simulink library "NetworksLib"  (Simulink 7.5)
settings: Solver=ode45  SolverMode=SingleTasking  StartTime=0.0  StopTime=10.0  RelTol=1e-3
undefined symbols (not defined in the file or in its folder): Others, SF, Sigmoid, to
libraries: simulink x3, NetworksLib x3, RateBasedLib x2, fuzblock x1, StimuliLib x1
settings Model: Creator=jpalma  LastModifiedBy=jpalma

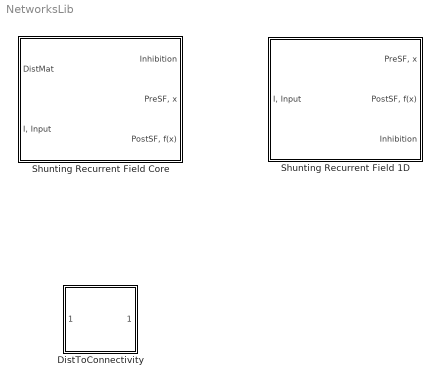
== system NetworksLib ==
  DistToConnectivity : Subsystem  mask{connectChoice=1-to-1, gaussWidth=1, gaussMean=0}
      mask prompts: gaussWidth "Gaussian Width"; gaussMean "Gaussian Mean"
      mask StyleString: popup(1-to-1|1-to-All|1-to-Others|Gaussian),edit,edit
      mask CallbackString:
      | maskStr = get_param(gcb,'MaskValues');
      | visibilitiesStr = {'on';'off';'off'};
      | if strcmp(maskStr{1},'Gaussian')
      |         visibilitiesStr(2) = {'on'};
      |         visibilitiesStr(3) = {'on'};
      | end
      | set_param(gcb,'MaskVisibilities',visibilitiesStr);||
      mask Display: image(imread('../libs/icons/Connect.jpg'),'center');
  Shunting Recurrent Field 1D : Subsystem  mask{signalFunction=Sigmoid-SF, threshold=0.3, thresholdSwitch=0, slope=9, asymptote=1, ground=0, A=0.1, B=1, fieldLength=10, ifCyclic=off, C=1, D=1, tau=1, inhibConnect=1-to-Others, inhibWidth=5, excitConnect=1-to-1, excitWidth=2}
      mask prompts: signalFunction "Signal Function Choice"; threshold "Threshold (SF)"; thresholdSwitch "Threshold of Switch (SF)"; slope "Slope (SF)"; asymptote "Asymptote (SF)"; ground "Ground (SF)"; A "A, Neuron Decay"; B "B, Neuron Shunting Max"; fieldLength "Field Length"; ifCyclic "Cyclic?"; C "C, Inhibitory Strength"; D "D, Excitatory Strength"; tau "tau, Time Constant"; inhibConnect "Inhibitory Connectivity"; inhibWidth "Inhibitory Width"; excitConnect "Excitatory Connectectivity"; excitWidth "Excitatory Width"
      mask init:
      | set_param([gcb '/Shunting Recurrent Field Core'], 'signalFunction', signalFunction);
      | set_param([gcb '/Shunting Recurrent Field Core'], 'threshold', threshold);
      | set_param([gcb '/Shunting Recurrent Field Core'], 'thresholdSwitch', thresholdSwitch);
      | set_param([gcb '/Shunting Recurrent Field Core'], 'slope', slope);
      | set_param([gcb '/Shunting Recurrent Field Core'], 'asymptote', asymptote);
      | set_param([gcb '/Shunting Recurrent Field Core'], 'ground', ground);
      | set_param([gcb '/Shunting Recurrent Field Core'], 'A', A);
      | set_param([gcb '/Shunting Recurrent Field Core'], 'B', B);
      | set_param([gcb '/Shunting Recurrent Field Core'], 'C', C);
      | set_param([gcb '/Shunting Recurrent Field Core'], 'D', D);
      | set_param([gcb '/Shunting Recurrent Field Core'], 'tau', tau);
      | set_param([gcb '/Shunting Recurrent Field Core'], 'inhibConnect', inhibConnect);
      | set_param([gcb '/Shunting Recurrent Field Core'], 'inhibWidth', inhibWidth);
      | set_param([gcb '/Shunting Recurrent Field Core'], 'excitConnect', excitConnect);
      | set_param([gcb '/Shunting Recurrent Field Core'], 'excitWidth', excitWidth);
      | set_param([gcb '/DistMatrix1D'], 'vectorLength', fieldLength);
      | set_param([gcb '/DistMatrix1D'], 'ifCyclic', ifCyclic);
      mask StyleString: popup(Linear-SF|Faster-SF|Slower-SF|Sigmoid-SF|Sigmoid-To-Linear-SF),edit,edit,edit,edit,edit,edit,edit,edit,checkbox,edit,edit,edit,popup(1-to-1|1-to-All|1-to-Others|Gaussian),edit,popup(1-to-1|1-to-All|1-to-Others|Gaussian),edit
      mask CallbackString:
      | maskStr = get_param(gcb,'MaskValues');
      | 
      | visibilitiesStr = {'on';'off';'off';'off';'off';'off';'on';'on'; ...
      |                    'on';'on';'on';'on';'on';'on';'off';'on';'off'};
      | if strcmp(maskStr{1},'Sigmoid-SF')
      |         visibilitiesStr(2) = {'on'};
      |         visibilitiesStr(4) = {'on'};
      |         visibilitiesStr(5) = {'on'};
      |         visibilitiesStr(6) = {'on'};
      | else if strcmp(maskStr{1},'Sigmoid-To-Linear-SF')
      |         visibilitiesStr(2) = {'on'};
      |         visibilitiesStr(3) = {'on'};
      |         visibilitiesStr(4) = {'on'};
      |         visibilitiesStr(5) = {'on'};
      |         visibilitiesStr(6) = {'on'};
      |     end
      | end
      | if strcmp(maskStr{14},'Gaussian')
      |         visibilitiesStr(15) = {'on'};
      | end
      | if strcmp(maskStr{16},'Gaussian')
      |         visibilitiesStr(17) = {'on'};
      | end
      | set_param(gcb,'MaskVisibilities',visibilitiesStr);
      | |||||||||||||maskStr = get_param(gcb,'MaskValues');
      | 
      | visibilitiesStr = {'on';'off';'off';'off';'off';'off';'on';'on'; ...
      |                    'on';'on';'on';'on';'on';'on';'off';'on';'off'};
      | if strcmp(maskStr{1},'Sigmoid-SF')
      |         visibilitiesStr(2) = {'on'};
      |         visibilitiesStr(4) = {'on'};
      |         visibilitiesStr(5) = {'on'};
      |         visibilitiesStr(6) = {'on'};
      | else if strcmp(maskStr{1},'Sigmoid-To-Linear-SF')
      |         visibilitiesStr(2) = {'on'};
      |         visibilitiesStr(3) = {'on'};
      |         visibilitiesStr(4) = {'on'};
      |         visibilitiesStr(5) = {'on'};
      |         visibilitiesStr(6) = {'on'};
      |     end
      | end
      | if strcmp(maskStr{14},'Gaussian')
      |         visibilitiesStr(15) = {'on'};
      | end
      | if strcmp(maskStr{16},'Gaussian')
      |         visibilitiesStr(17) = {'on'};
      | end
      | set_param(gcb,'MaskVisibilities',visibilitiesStr);||maskStr = get_param(gcb,'MaskValues');
      | 
      | visibilitiesStr = {'on';'off';'off';'off';'off';'off';'on';'on'; ...
      |                    'on';'on';'on';'on';'on';'on';'off';'on';'off'};
      | if strcmp(maskStr{1},'Sigmoid-SF')
      |         visibilitiesStr(2) = {'on'};
      |         visibilitiesStr(4) = {'on'};
      |         visibilitiesStr(5) = {'on'};
      |         visibilitiesStr(6) = {'on'};
      | else if strcmp(maskStr{1},'Sigmoid-To-Linear-SF')
      |         visibilitiesStr(2) = {'on'};
      |         visibilitiesStr(3) = {'on'};
      |         visibilitiesStr(4) = {'on'};
      |         visibilitiesStr(5) = {'on'};
      |         visibilitiesStr(6) = {'on'};
      |     end
      | end
      | if strcmp(maskStr{14},'Gaussian')
      |         visibilitiesStr(15) = {'on'};
      | end
      | if strcmp(maskStr{16},'Gaussian')
      |         visibilitiesStr(17) = {'on'};
      | end
      | set_param(gcb,'MaskVisibilities',visibilitiesStr);|
      mask Display: image(imread('../libs/icons/Networks.jpg'),'center');
  Shunting Recurrent Field Core : Subsystem  mask{signalFunction=Sigmoid-SF, threshold=0.3, thresholdSwitch=0, slope=9, asymptote=1, ground=0, A=0.1, B=1, C=1, D=1, tau=1, inhibConnect=1-to-Others, inhibWidth=5, excitConnect=1-to-1, excitWidth=2}
      mask prompts: signalFunction "Signal Function Choice"; threshold "Threshold (SF)"; thresholdSwitch "Threshold of Switch (SF)"; slope "Slope (SF)"; asymptote "Asymptote (SF)"; ground "Gound (SF)"; A "A, Neuron Decay"; B "B, Neuron Shunting Max"; C "C, Inhibitory Strength"; D "D, Excitatory Strength"; tau "tau, Time Constant"; inhibConnect "Inhibitory Connectivity"; inhibWidth "Inhibitory Width"; excitConnect "Excitatory Connectivity"; excitWidth "Excitatory Width"
      mask init:
      | set_param([gcb '/Signal Function'], 'BlockChoice', signalFunction);
      | if(strcmp(signalFunction,'Sigmoid-SF'))
      |    maskStr = get_param([gcb '/Signal Function/' signalFunction],'MaskValues');
      |    maskStr{1} = threshold;
      |    maskStr{2} = slope;
      |    maskStr{3} = asymptote;
      |    maskStr{4} = ground;
      |    set_param([gcb '/Signal Function/' signalFunction], 'MaskValues', maskStr);
      | end
      | if(strcmp(signalFunction,'Sigmoid-To-Linear-SF'))
      |    maskStr = get_param([gcb '/Signal Function/' signalFunction],'MaskValues');
      |    maskStr{1} = threshold;
      |    maskStr{2} = thresholdSwitch;
      |    maskStr{3} = slope;
      |    maskStr{4} = asymptote;
      |    maskStr{5} = ground;
      |    set_param([gcb '/Signal Function/' signalFunction], 'MaskValues', maskStr);
      | end
      | set_param([gcb '/InhibConnectivity'], 'connectChoice', inhibConnect);
      | set_param([gcb '/InhibConnectivity'], 'gaussWidth', inhibWidth);
      | set_param([gcb '/InhibConnectivity'], 'gaussMean', '0');
      | set_param([gcb '/ExcitConnectivity'], 'connectChoice', excitConnect);
      | set_param([gcb '/ExcitConnectivity'], 'gaussWidth', excitWidth);
      | set_param([gcb '/ExcitConnectivity'], 'gaussMean', '0');
      mask StyleString: popup(Linear-SF|Faster-SF|Slower-SF|Sigmoid-SF|Sigmoid-To-Linear-SF),edit,edit,edit,edit,edit,edit,edit,edit,edit,edit,popup(1-to-1|1-to-All|1-to-Others|Gaussian),edit,popup(1-to-1|1-to-All|1-to-Others|Gaussian),edit
      mask CallbackString:
      | maskStr = get_param(gcb,'MaskValues');
      | 
      | visibilitiesStr = {'on';'off';'off';'off';'off';'off';'on';'on'; ...
      |                    'on';'on';'on';'on';'off';'on';'off'};
      | if strcmp(maskStr{1},'Sigmoid-SF')
      |         visibilitiesStr(2) = {'on'};
      |         visibilitiesStr(4) = {'on'};
      |         visibilitiesStr(5) = {'on'};
      |         visibilitiesStr(6) = {'on'};
      | else if strcmp(maskStr{1},'Sigmoid-To-Linear-SF')
      |         visibilitiesStr(2) = {'on'};
      |         visibilitiesStr(3) = {'on'};
      |         visibilitiesStr(4) = {'on'};
      |         visibilitiesStr(5) = {'on'};
      |         visibilitiesStr(6) = {'on'};
      |     end
      | end
      | if strcmp(maskStr{12},'Gaussian')
      |         visibilitiesStr(13) = {'on'};
      | end
      | if strcmp(maskStr{14},'Gaussian')
      |         visibilitiesStr(15) = {'on'};
      | end
      | set_param(gcb,'MaskVisibilities',visibilitiesStr);
      | |||||||||||maskStr = get_param(gcb,'MaskValues');
      | 
      | visibilitiesStr = {'on';'off';'off';'off';'off';'off';'on';'on'; ...
      |                    'on';'on';'on';'on';'off';'on';'off'};
      | if strcmp(maskStr{1},'Sigmoid-SF')
      |         visibilitiesStr(2) = {'on'};
      |         visibilitiesStr(4) = {'on'};
      |         visibilitiesStr(5) = {'on'};
      |         visibilitiesStr(6) = {'on'};
      | else if strcmp(maskStr{1},'Sigmoid-To-Linear-SF')
      |         visibilitiesStr(2) = {'on'};
      |         visibilitiesStr(3) = {'on'};
      |         visibilitiesStr(4) = {'on'};
      |         visibilitiesStr(5) = {'on'};
      |         visibilitiesStr(6) = {'on'};
      |     end
      | end
      | if strcmp(maskStr{12},'Gaussian')
      |         visibilitiesStr(13) = {'on'};
      | end
      | if strcmp(maskStr{14},'Gaussian')
      |         visibilitiesStr(15) = {'on'};
      | end
      | set_param(gcb,'MaskVisibilities',visibilitiesStr);
      | 
      | ||maskStr = get_param(gcb,'MaskValues');
      | 
      | visibilitiesStr = {'on';'off';'off';'off';'off';'off';'on';'on'; ...
      |                    'on';'on';'on';'on';'off';'on';'off'};
      | if strcmp(maskStr{1},'Sigmoid-SF')
      |         visibilitiesStr(2) = {'on'};
      |         visibilitiesStr(4) = {'on'};
      |         visibilitiesStr(5) = {'on'};
      |         visibilitiesStr(6) = {'on'};
      | else if strcmp(maskStr{1},'Sigmoid-To-Linear-SF')
      |         visibilitiesStr(2) = {'on'};
      |         visibilitiesStr(3) = {'on'};
      |         visibilitiesStr(4) = {'on'};
      |         visibilitiesStr(5) = {'on'};
      |         visibilitiesStr(6) = {'on'};
      |     end
      | end
      | if strcmp(maskStr{12},'Gaussian')
      |         visibilitiesStr(13) = {'on'};
      | end
      | if strcmp(maskStr{14},'Gaussian')
      |         visibilitiesStr(15) = {'on'};
      | end
      | set_param(gcb,'MaskVisibilities',visibilitiesStr);
      | 
      | |
      mask Display: image(imread('../libs/icons/Networks.jpg'),'center');

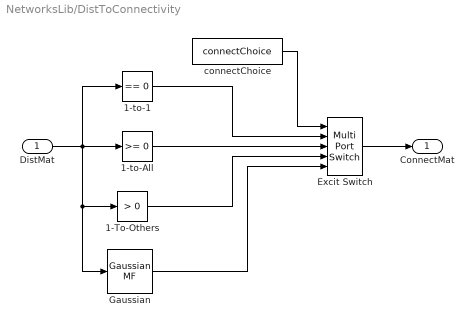
== system NetworksLib/DistToConnectivity ==
  DistMat : Inport
  1-To-Others : simulink/Logic and Bit Operations/Compare To Zero  SystemSampleTime=-1  relop=>  LogicOutDataTypeMode=uint8  ZeroCross=off
  1-to-1 : simulink/Logic and Bit Operations/Compare To Zero  SystemSampleTime=-1  relop===  LogicOutDataTypeMode=uint8  ZeroCross=off
  1-to-All : simulink/Logic and Bit Operations/Compare To Zero  SystemSampleTime=-1  relop=>=  LogicOutDataTypeMode=uint8  ZeroCross=off
  Excit Switch : MultiPortSwitch  Inputs=4  zeroidx=off  OutDataType=sfix(16)  OutScaling=2^0
  Gaussian : fuzblock/Membership  Functions/Gaussian MF  SystemSampleTime=-1  sigma=gaussWidth  mu=gaussMean
  connectChoice : Constant  Value=connectChoice  OutDataType=sfix(16)  OutScaling=2^0
  ConnectMat : Outport
  wires:
  DistMat/1 -> Gaussian/1, 1-To-Others/1, 1-to-All/1, 1-to-1/1
  Excit Switch/1 -> ConnectMat/1
  1-to-1/1 -> Excit Switch/2
  connectChoice/1 -> Excit Switch/1
  1-to-All/1 -> Excit Switch/3
  1-To-Others/1 -> Excit Switch/4
  Gaussian/1 -> Excit Switch/5

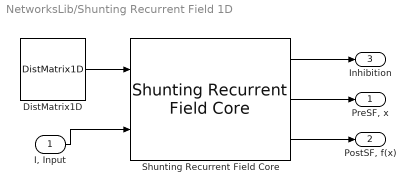
== system NetworksLib/Shunting Recurrent Field 1D ==
  "I, Input" : Inport
  DistMatrix1D : StimuliLib/DistMatrix1D  SystemSampleTime=-1  vectorLength=10  ifCyclic=off
  Shunting Recurrent Field Core : NetworksLib/Shunting Recurrent Field Core  SystemSampleTime=-1  signalFunction=Sigmoid-SF  threshold=0.3  thresholdSwitch=0  slope=9  asymptote=1  ground=0  A=0.1  B=1  C=1  D=1  tau=1  inhibConnect=1-to-Others  inhibWidth=5  excitConnect=1-to-1  excitWidth=2
  "PreSF, x" : Outport
  "PostSF, f(x)" : Outport  Port=2
  Inhibition : Outport  Port=3
  wires:
  Shunting Recurrent Field Core/1 -> Inhibition/1
  DistMatrix1D/1 -> Shunting Recurrent Field Core/1
  Shunting Recurrent Field Core/3 -> "PostSF, f(x)"/1
  Shunting Recurrent Field Core/2 -> "PreSF, x"/1
  "I, Input"/1 -> Shunting Recurrent Field Core/2

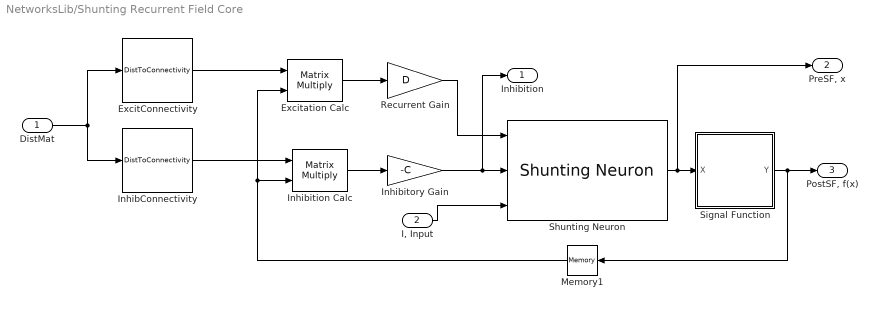
== system NetworksLib/Shunting Recurrent Field Core ==
  DistMat : Inport
  "I, Input" : Inport  Port=2
  ExcitConnectivity : NetworksLib/DistToConnectivity  SystemSampleTime=-1  connectChoice=1-to-1  gaussWidth=2  gaussMean=0
  Excitation Calc : Product  Multiplication=Matrix(*)  OutDataType=sfix(16)  OutScaling=2^0
  InhibConnectivity : NetworksLib/DistToConnectivity  SystemSampleTime=-1  connectChoice=1-to-Others  gaussWidth=5  gaussMean=0
  Inhibition Calc : Product  Multiplication=Matrix(*)  OutDataType=sfix(16)  OutScaling=2^0
  Inhibitory Gain : Gain  Gain=-C  ParameterDataType=sfix(16)  ParameterScaling=2^0  OutDataType=sfix(16)  OutScaling=2^0
  Memory1 : Memory
  Recurrent Gain : Gain  Gain=D  ParameterDataType=sfix(16)  ParameterScaling=2^0  OutDataType=sfix(16)  OutScaling=2^0
  Shunting Neuron : RateBasedLib/Shunting Neuron  SystemSampleTime=-1  A=A  B=B  tau=tau
  Signal Function : Subsystem  BlockChoice=Sigmoid-SF
      settings: AttributesFormatString=%<BlockChoice>  TemplateBlock=RateBasedLib/Signal Function  MemberBlocks=Faster-SF,Linear-SF,Sigmoid-SF,Sigmoid-To-Linear-SF,Slower-SF
  Inhibition : Outport
  "PreSF, x" : Outport  Port=2
  "PostSF, f(x)" : Outport  Port=3
  wires:
  Excitation Calc/1 -> Recurrent Gain/1
  Inhibition Calc/1 -> Inhibitory Gain/1
  Memory1/1 -> Inhibition Calc/2, Excitation Calc/2
  ExcitConnectivity/1 -> Excitation Calc/1
  Signal Function/1(Y) -> Memory1/1, "PostSF, f(x)"/1
  Shunting Neuron/1 -> Signal Function/1(X), "PreSF, x"/1
  Inhibitory Gain/1 -> Shunting Neuron/2, Inhibition/1
  "I, Input"/1 -> Shunting Neuron/3
  DistMat/1 -> InhibConnectivity/1, ExcitConnectivity/1
  InhibConnectivity/1 -> Inhibition Calc/1
  Recurrent Gain/1 -> Shunting Neuron/1

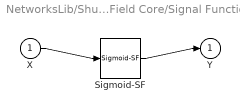
== system NetworksLib/Shunting Recurrent Field Core/Signal Function ==
  X : Inport
  Sigmoid-SF : RateBasedLib/Sigmoid-SF  SystemSampleTime=-1  threshold=0.3  slope=9  asymptote=1  ground=0
  Y : Outport
  wires:
  X/1 -> Sigmoid-SF/1
  Sigmoid-SF/1 -> Y/1
